simulink model "FREE_DRIFT"  (R2020b)
settings: Solver=ode4  StartTime=0.0  StopTime=500  FixedStep=Dt  RelTol=1e-3
values from neighbouring files (symbols this model uses):
  alpha = 0.01    [INPUTS_GRUPPO20.m]
  e_ss = 0.02    [INPUTS_GRUPPO20.m]
  enable_drag = 1    [INPUTS_GRUPPO20.m]
  enable_J2 = 1    [INPUTS_GRUPPO20.m]
  enable_Mgrav = 1    [INPUTS_GRUPPO20.m]
  enable_PD = 1    [INPUTS_GRUPPO20.m]
  enable_SMC = 0    [INPUTS_GRUPPO20.m]
  F_D = -1/2*rho*CD*A*Vx^2    (= -3.88125057814e-05)    [INPUTS_GRUPPO20.m]
  FJ2 = -3*J2*m_c0*mu*r_E^2/(2*r^4)    (= -0.00149705073945)    [INPUTS_GRUPPO20.m]
  gmax = 0.005    [INPUTS_GRUPPO20.m]
  INV_ZZZ = pinv(ZZZ)    [INPUTS_GRUPPO20.m]
  invJ = inv(J)    [INPUTS_GRUPPO20.m]
  J = J0    [INPUTS_GRUPPO20.m]
  kd = d*eye(3)    [INPUTS_GRUPPO20.m]
  kp1 = k*eye(3)    [INPUTS_GRUPPO20.m]
  Kr = 1    [INPUTS_GRUPPO20.m]
  lambda = 0.03    [INPUTS_GRUPPO20.m]
  m_c0 = 120    [INPUTS_GRUPPO20.m]
  omega = (mu/r^3)^0.5    (= 0.00113136572666)    [INPUTS_GRUPPO20.m]
  p_RW = 1    [INPUTS_GRUPPO20.m]
  Pos0 = Pos_RB(end,:)'    [INPUTS_GRUPPO20.m]
  q0_0 = Q_RB(end,1)'    [INPUTS_GRUPPO20.m]
  q_des = [1 0 0 0]'    [INPUTS_GRUPPO20.m]
  qv_0 = Q_RB(end,2:4)'    [INPUTS_GRUPPO20.m]
  tau_RW = 1.5645e-2    (= 0.015645)    [INPUTS_GRUPPO20.m]
  Vel0 = Vel_RB(end,:)'    [INPUTS_GRUPPO20.m]
  wb_0 = wb_RB(end,:)'    [INPUTS_GRUPPO20.m]
  X0_H = -10250    [INPUTS_GRUPPO20.m]
  ZZZ = [cos(B)    0      -cos(B)    0 ... (first row only)    [INPUTS_GRUPPO20.m]
undefined symbols (not defined in the file or in its folder): magnitude
libraries: vrlib x3, aerolibutil x1, sharedtransform x1
settings Model: Creator=Beniamino  LastModifiedBy=Beniamino

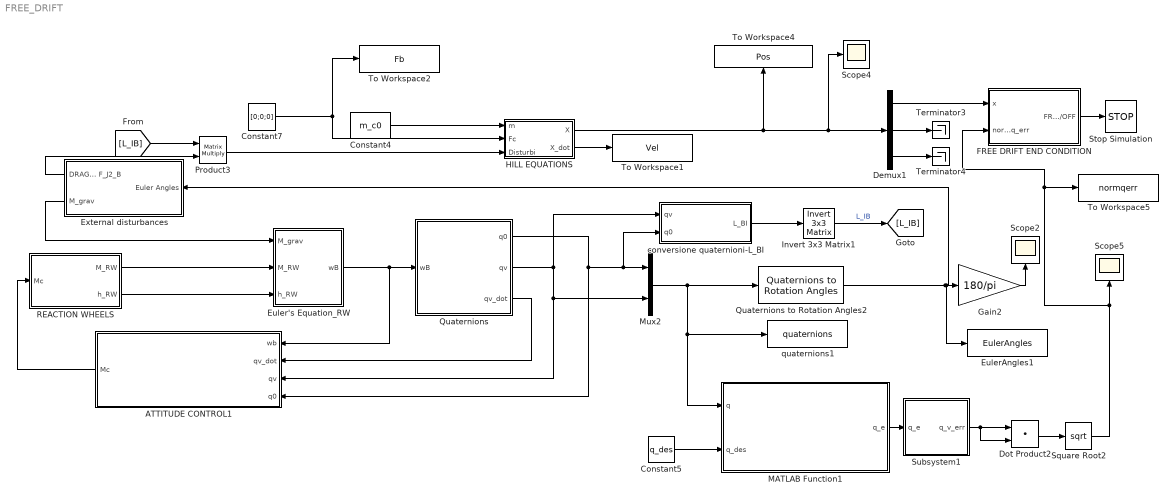
== system FREE_DRIFT ==
  ATTITUDE CONTROL1 : Subsystem
  Constant4 : Constant  Value=m_c0
  Constant5 : Constant  Value=q_des
  Constant7 : Constant  Value=[0;0;0]
  Demux1 : Demux  Outputs=3
  Dot Product2 : DotProduct  InputSameDT=on  OutDataTypeStr=Inherit: Inherit via internal rule
  Euler's Equation_RW : Subsystem
  EulerAngles1 : ToWorkspace  VariableName=EulerAngles  SampleTime=-1
  External disturbances : Subsystem
  FREE DRIFT END CONDITION : Subsystem
  Gain2 : Gain  Gain=180/pi
  HILL EQUATIONS : Subsystem
  Invert 3x3 Matrix1 : aerolibutil/Invert  3x3 Matrix
  MATLAB Function1 : MATLAB Function  TreatAsAtomicUnit=on
  Mux2 : Mux  Inputs=2
  Product3 : Product  Multiplication=Matrix(*)
  Quaternions : Subsystem
  Quaternions to Rotation Angles2 : sharedtransform/Quaternions to Rotation Angles  rotationOrder=ZYX  aMode=aMode
      settings: SourceProductBaseCode=AE,PW,MT,UV,VE,VP
  REACTION WHEELS : Subsystem
  Scope2 : Scope
  Scope4 : Scope
  Scope5 : Scope
  Square Root2 : Sqrt  SaturateOnIntegerOverflow=on
  Stop Simulation : Stop
  Subsystem1 : Subsystem
  Terminator3 : Terminator
  Terminator4 : Terminator
  To Workspace1 : ToWorkspace  VariableName=Vel  SampleTime=-1
  To Workspace2 : ToWorkspace  VariableName=Fb  SampleTime=-1
  To Workspace4 : ToWorkspace  VariableName=Pos  SampleTime=-1
  To Workspace5 : ToWorkspace  VariableName=normqerr  SampleTime=-1
  conversione quaternioni-L_BI : Subsystem
  quaternions1 : ToWorkspace  VariableName=quaternions  SampleTime=-1
  wires:
  External disturbances/2(M_grav) -> Euler's Equation_RW/1(M_grav)
  [L_IB] -> Product3/1
  Quaternions to Rotation Angles2/1 -> External disturbances/1(Euler Angles), EulerAngles1/1, Gain2/1
  REACTION WHEELS/2("h_RW ") -> Euler's Equation_RW/3(h_RW)
  Invert 3x3 Matrix1/1 -> [L_IB]  "L_IB"
  Product3/1 -> HILL EQUATIONS/3(Disturbi)
  Quaternions/1(q0) -> ATTITUDE CONTROL1/4(q0), Mux2/1, conversione quaternioni-L_BI/2(q0)
  Constant5/1 -> MATLAB Function1/2(q_des)
  Quaternions/3(qv_dot) -> ATTITUDE CONTROL1/2(qv_dot)
  External disturbances/1(DRAG_B + F_J2_B) -> Product3/2
  REACTION WHEELS/1(M_RW) -> Euler's Equation_RW/2(M_RW)
  Euler's Equation_RW/1(wB) -> ATTITUDE CONTROL1/1(wb), Quaternions/1(wB)
  MATLAB Function1/1(q_e) -> Subsystem1/1(q_e)
  Gain2/1 -> Scope2/1
  Subsystem1/1(q_v_err) -> Dot Product2/2, Dot Product2/1
  Quaternions/2(qv) -> ATTITUDE CONTROL1/3(qv), Mux2/2, conversione quaternioni-L_BI/1(qv)
  Mux2/1 -> Quaternions to Rotation Angles2/1, MATLAB Function1/1(q), quaternions1/1
  ATTITUDE CONTROL1/1(Mc) -> REACTION WHEELS/1(Mc)
  conversione quaternioni-L_BI/1(L_BI) -> Invert 3x3 Matrix1/1
  Dot Product2/1 -> Square Root2/1
  Constant7/1 -> HILL EQUATIONS/2(Fc), To Workspace2/1
  HILL EQUATIONS/2(X_dot) -> To Workspace1/1
  HILL EQUATIONS/1(X) -> Scope4/1, Demux1/1, To Workspace4/1
  Demux1/1 -> FREE DRIFT END CONDITION/1(x)
  Demux1/2 -> Terminator3/1
  Demux1/3 -> Terminator4/1
  Square Root2/1 -> To Workspace5/1, FREE DRIFT END CONDITION/2(norma q_err), Scope5/1
  FREE DRIFT END CONDITION/1(FREE DRIFT ON/OFF) -> Stop Simulation/1
  Constant4/1 -> HILL EQUATIONS/1(m)

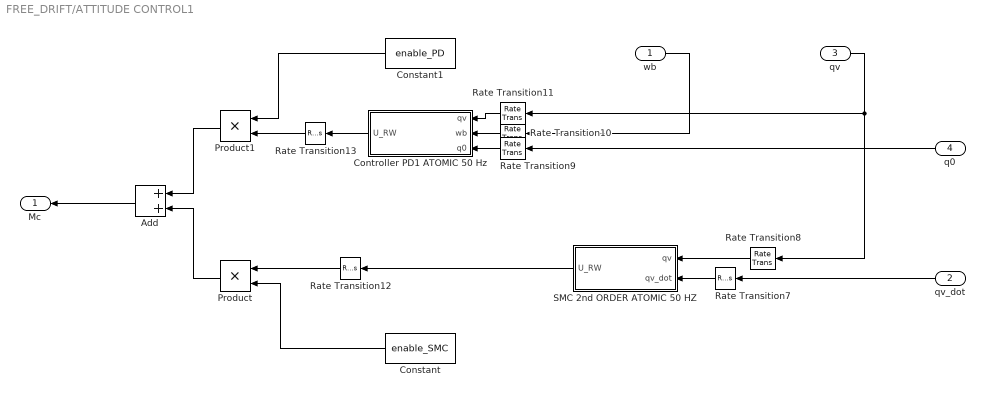
== system FREE_DRIFT/ATTITUDE CONTROL1 ==
  wb : Inport
  qv_dot : Inport  Port=2
  qv : Inport  Port=3
  q0 : Inport  Port=4
  Add : Sum
  Constant : Constant  Value=enable_SMC
  Constant1 : Constant  Value=enable_PD
  Controller PD1 ATOMIC 50 Hz : Subsystem  TreatAsAtomicUnit=on  SystemSampleTime=0.02
  Product : Product
  Product1 : Product
  Rate Transition{7..11} (5 alike) : RateTransition  OutPortSampleTime=Dt_con
  Rate Transition12 : RateTransition  OutPortSampleTime=Dt
  Rate Transition13 : RateTransition  OutPortSampleTime=Dt
  SMC 2nd ORDER ATOMIC 50 HZ : Subsystem  TreatAsAtomicUnit=on  SystemSampleTime=0.02
  Mc : Outport
  wires:
  Add/1 -> Mc/1
  qv_dot/1 -> Rate Transition7/1
  q0/1 -> Rate Transition9/1
  SMC 2nd ORDER ATOMIC 50 HZ/1(U_RW) -> Rate Transition12/1
  Controller PD1 ATOMIC 50 Hz/1(U_RW) -> Rate Transition13/1
  Rate Transition8/1 -> SMC 2nd ORDER ATOMIC 50 HZ/1(qv)
  wb/1 -> Rate Transition10/1
  Rate Transition7/1 -> SMC 2nd ORDER ATOMIC 50 HZ/2(qv_dot)
  Rate Transition10/1 -> Controller PD1 ATOMIC 50 Hz/2(wb)
  Rate Transition11/1 -> Controller PD1 ATOMIC 50 Hz/1(qv)
  qv/1 -> Rate Transition11/1, Rate Transition8/1
  Rate Transition9/1 -> Controller PD1 ATOMIC 50 Hz/3(q0)
  Rate Transition12/1 -> Product/1
  Constant/1 -> Product/2
  Rate Transition13/1 -> Product1/2
  Constant1/1 -> Product1/1
  Product1/1 -> Add/1
  Product/1 -> Add/2

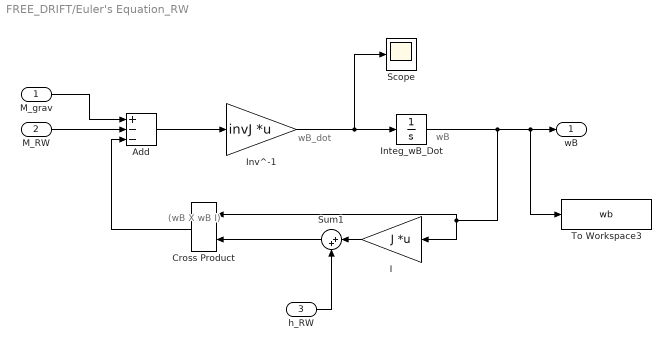
== system FREE_DRIFT/Euler's Equation_RW ==
  note: (wB X wB I)
  note: wB
  note: wB_dot
  M_grav : Inport
  M_RW : Inport  Port=2
  h_RW : Inport  Port=3
  Add : Sum  Inputs=+--
  Cross Product : vrlib/Utilities/Cross Product
  I : Gain  Gain=J  Multiplication=Matrix(K*u)
  Integ_wB_Dot : Integrator  InitialCondition=wb_0
  Inv^-1 : Gain  Gain=invJ  Multiplication=Matrix(K*u)
  Scope : Scope
  Sum1 : Sum  Inputs=|++
  To Workspace3 : ToWorkspace  VariableName=wb  SampleTime=-1
  wB : Outport  VectorParamsAs1DForOutWhenUnconnected=off
  wires:
  M_grav/1 -> Add/1
  Sum1/1 -> Cross Product/2
  h_RW/1 -> Sum1/2
  Integ_wB_Dot/1 -> To Workspace3/1, wB/1, Cross Product/1, I/1
  I/1 -> Sum1/1
  M_RW/1 -> Add/2
  Add/1 -> Inv^-1/1
  Inv^-1/1 -> Scope/1, Integ_wB_Dot/1
  Cross Product/1 -> Add/3

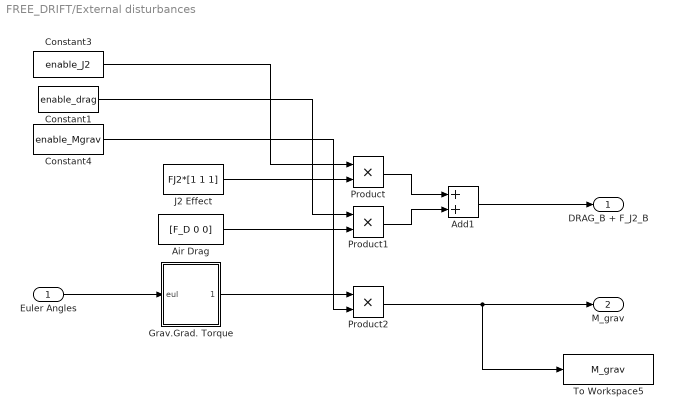
== system FREE_DRIFT/External disturbances ==
  Euler Angles : Inport
  Add1 : Sum
  Air Drag : Constant  Value=[F_D 0 0]
  Constant1 : Constant  Value=enable_drag
  Constant3 : Constant  Value=enable_J2
  Constant4 : Constant  Value=enable_Mgrav
  Grav.Grad. Torque : Subsystem
  J2 Effect : Constant  Value=FJ2*[1 1 1]
  Product : Product
  Product1 : Product
  Product2 : Product
  To Workspace5 : ToWorkspace  VariableName=M_grav  SampleTime=-1
  DRAG_B + F_J2_B : Outport
  M_grav : Outport  Port=2
  wires:
  Grav.Grad. Torque/1(M_grav) -> Product2/1
  Euler Angles/1 -> Grav.Grad. Torque/1(eul)
  Add1/1 -> DRAG_B + F_J2_B/1
  Constant3/1 -> Product/1
  J2 Effect/1 -> Product/2
  Constant1/1 -> Product1/1
  Air Drag/1 -> Product1/2
  Constant4/1 -> Product2/2
  Product/1 -> Add1/1
  Product1/1 -> Add1/2
  Product2/1 -> To Workspace5/1, M_grav/1

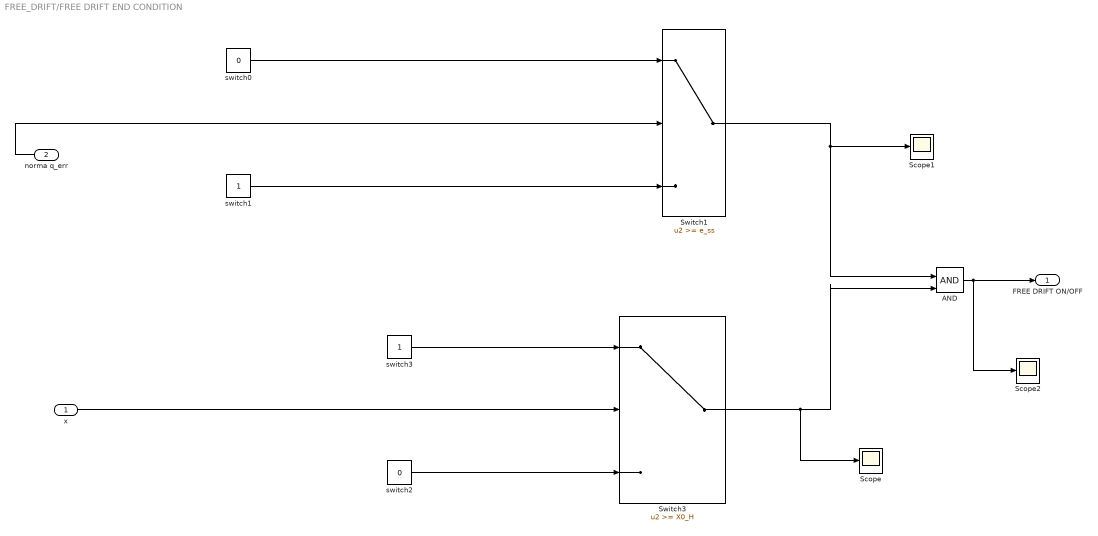
== system FREE_DRIFT/FREE DRIFT END CONDITION ==
  x : Inport
  norma q_err : Inport  Port=2
  AND : Logic  IconShape=distinctive  AllPortsSameDT=off  OutDataTypeStr=boolean
  Scope : Scope
  Scope1 : Scope
  Scope2 : Scope
  Switch1 : Switch  Threshold=e_ss
  Switch3 : Switch  Threshold=X0_H
  switch0 : Constant  Value=0
  switch1 : Constant
  switch2 : Constant  Value=0
  switch3 : Constant
  FREE DRIFT ON/OFF : Outport
  wires:
  norma q_err/1 -> Switch1/2
  Switch1/1 -> Scope1/1, AND/1
  switch0/1 -> Switch1/1
  switch2/1 -> Switch3/3
  Switch3/1 -> Scope/1, AND/2
  switch3/1 -> Switch3/1
  AND/1 -> Scope2/1, FREE DRIFT ON/OFF/1
  switch1/1 -> Switch1/3
  x/1 -> Switch3/2

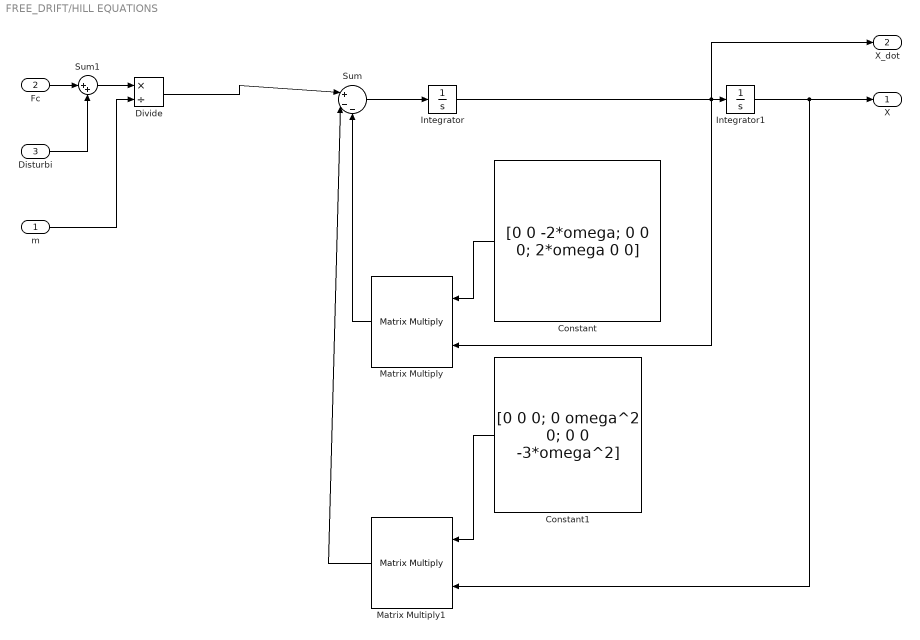
== system FREE_DRIFT/HILL EQUATIONS ==
  m : Inport
  Fc : Inport  Port=2
  Disturbi : Inport  Port=3
  Constant : Constant  Value=[0 0 -2*omega; 0 0 0; 2*omega 0 0]
  Constant1 : Constant  Value=[0 0 0; 0 omega^2 0; 0 0 -3*omega^2]
  Divide : Product  Inputs=*/
  Integrator : Integrator  InitialCondition=Vel0
  Integrator1 : Integrator  InitialCondition=Pos0
  Matrix Multiply : Product  Multiplication=Matrix(*)
  Matrix Multiply1 : Product  Multiplication=Matrix(*)
  Sum : Sum  Inputs=|+--
  Sum1 : Sum  Inputs=|++
  X : Outport
  X_dot : Outport  Port=2
  wires:
  Constant/1 -> Matrix Multiply/1
  Sum1/1 -> Divide/1
  Disturbi/1 -> Sum1/2
  Integrator/1 -> Integrator1/1, X_dot/1, Matrix Multiply/2
  Fc/1 -> Sum1/1
  m/1 -> Divide/2
  Matrix Multiply1/1 -> Sum/2
  Matrix Multiply/1 -> Sum/3
  Constant1/1 -> Matrix Multiply1/1
  Integrator1/1 -> Matrix Multiply1/2, X/1
  Sum/1 -> Integrator/1
  Divide/1 -> Sum/1

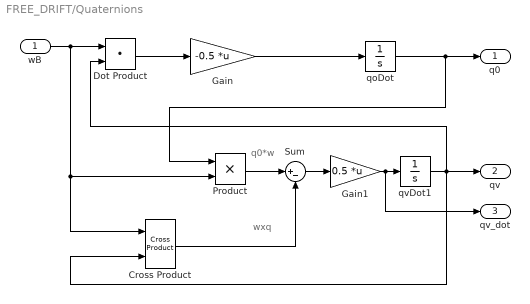
== system FREE_DRIFT/Quaternions ==
  note: wxq
  note: q0*w
  wB : Inport
  Cross Product : vrlib/Utilities/Cross Product
  Dot Product : DotProduct  InputSameDT=on  OutDataTypeStr=Inherit: Inherit via internal rule
  Gain : Gain  Gain=-0.5  Multiplication=Matrix(K*u)
  Gain1 : Gain  Gain=0.5  Multiplication=Matrix(K*u)
  Product : Product  RndMeth=Zero
  Sum : Sum  Inputs=|+-
  qoDot : Integrator  InitialCondition=q0_0
  qvDot1 : Integrator  InitialCondition=qv_0
  q0 : Outport  VectorParamsAs1DForOutWhenUnconnected=off
  qv : Outport  Port=2  VectorParamsAs1DForOutWhenUnconnected=off
  qv_dot : Outport  Port=3  VectorParamsAs1DForOutWhenUnconnected=off
  wires:
  qoDot/1 -> q0/1, Product/1
  qvDot1/1 -> Cross Product/2, qv/1, Dot Product/2
  wB/1 -> Cross Product/1, Product/2, Dot Product/1
  Dot Product/1 -> Gain/1
  Gain/1 -> qoDot/1
  Product/1 -> Sum/1
  Cross Product/1 -> Sum/2
  Sum/1 -> Gain1/1
  Gain1/1 -> qvDot1/1, qv_dot/1

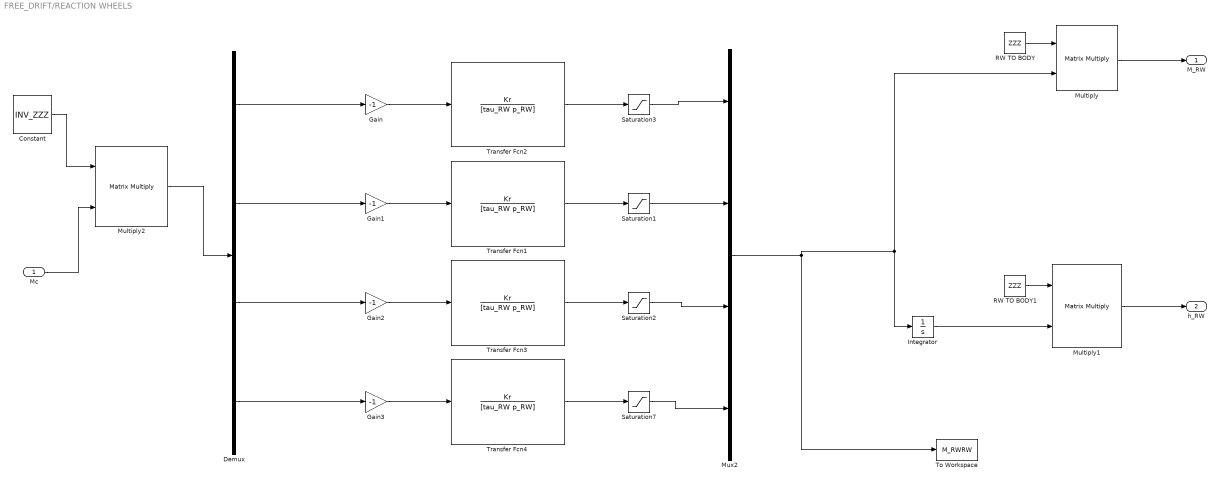
== system FREE_DRIFT/REACTION WHEELS ==
  Mc : Inport
  Constant : Constant  Value=INV_ZZZ
  Demux : Demux
  Gain{,1..3} (4 alike) : Gain  Gain=-1
  Integrator : Integrator
  Multiply : Product  Multiplication=Matrix(*)
  Multiply1 : Product  Multiplication=Matrix(*)
  Multiply2 : Product  Multiplication=Matrix(*)
  Mux2 : Mux
  RW TO BODY : Constant  Value=ZZZ
  RW TO BODY1 : Constant  Value=ZZZ
  Saturation{1..3,7} (4 alike) : Saturate  UpperLimit=gmax  LowerLimit=-gmax
  To Workspace : ToWorkspace  VariableName=M_RWRW  SampleTime=-1
  Transfer Fcn{1..4} (4 alike) : TransferFcn  Numerator=Kr  Denominator=[tau_RW p_RW]
  M_RW : Outport  VectorParamsAs1DForOutWhenUnconnected=off
  "h_RW " : Outport  Port=2  VectorParamsAs1DForOutWhenUnconnected=off
  wires:
  Mc/1 -> Multiply2/2
  Multiply/1 -> M_RW/1
  Demux/1 -> Gain/1
  Demux/2 -> Gain1/1
  Demux/3 -> Gain2/1
  Gain/1 -> Transfer Fcn2/1
  Gain1/1 -> Transfer Fcn1/1
  Gain2/1 -> Transfer Fcn3/1
  Multiply1/1 -> "h_RW "/1
  Demux/4 -> Gain3/1
  Gain3/1 -> Transfer Fcn4/1
  RW TO BODY/1 -> Multiply/1
  RW TO BODY1/1 -> Multiply1/1
  Constant/1 -> Multiply2/1
  Multiply2/1 -> Demux/1
  Transfer Fcn4/1 -> Saturation7/1
  Mux2/1 -> To Workspace/1, Multiply/2, Integrator/1
  Integrator/1 -> Multiply1/2
  Saturation7/1 -> Mux2/4
  Transfer Fcn3/1 -> Saturation2/1
  Saturation2/1 -> Mux2/3
  Transfer Fcn1/1 -> Saturation1/1
  Saturation1/1 -> Mux2/2
  Transfer Fcn2/1 -> Saturation3/1
  Saturation3/1 -> Mux2/1

== system FREE_DRIFT/Subsystem1 ==
  q_e : Inport
  Demux : Demux
  Mux1 : Mux  Inputs=3
  Terminator : Terminator
  q_v_err : Outport  VectorParamsAs1DForOutWhenUnconnected=off
  wires:
  Demux/3 -> Mux1/2
  Demux/2 -> Mux1/1
  Demux/4 -> Mux1/3
  Demux/1 -> Terminator/1
  q_e/1 -> Demux/1
  Mux1/1 -> q_v_err/1

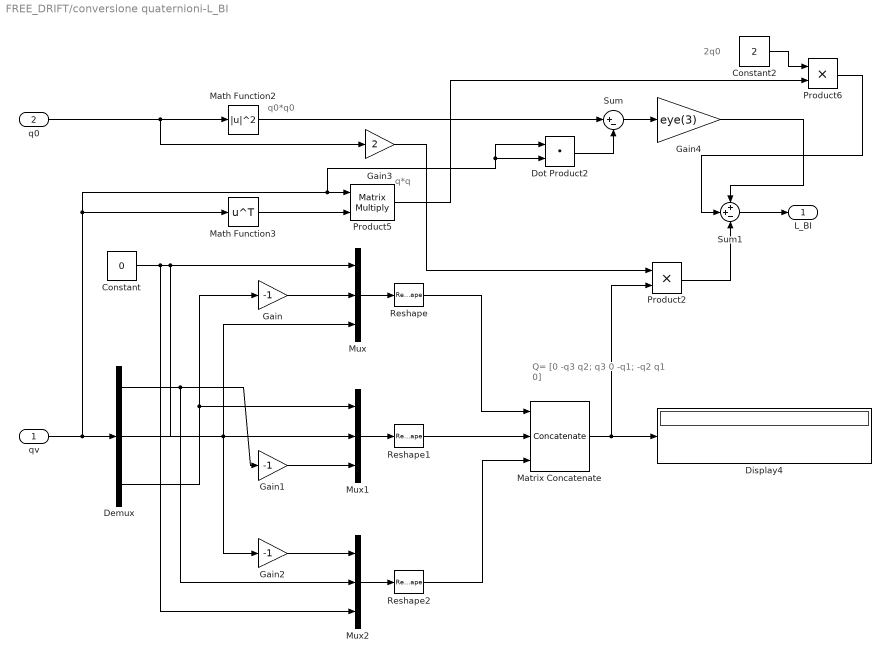
== system FREE_DRIFT/conversione quaternioni-L_BI ==
  note: Q= [0 -q3 q2;
      | 	q3 0 -q1;
      | 	-q2 q1 0]
  note: 2q0
  note: q*q
  note: q0*q0
  qv : Inport
  q0 : Inport  Port=2
  Constant : Constant  Value=0
  Constant2 : Constant  Value=2
  Demux : Demux  Outputs=3
  Display4 : Display
  Dot Product2 : DotProduct  InputSameDT=on  OutDataTypeStr=Inherit: Inherit via internal rule
  Gain : Gain  Gain=-1
  Gain1 : Gain  Gain=-1
  Gain2 : Gain  Gain=-1
  Gain3 : Gain  Gain=2
  Gain4 : Gain  Gain=eye(3)
  Math Function2 : Math  Operator=magnitude^2  SignedPower=on  SaturateOnIntegerOverflow=on
  Math Function3 : Math  Operator=transpose  SignedPower=on  SaturateOnIntegerOverflow=on
  Matrix Concatenate : Concatenate  NumInputs=3  Mode=Multidimensional array
  Mux : Mux  Inputs=3
  Mux1 : Mux  Inputs=3
  Mux2 : Mux  Inputs=3
  Product2 : Product  RndMeth=Zero
  Product5 : Product  Multiplication=Matrix(*)
  Product6 : Product
  Reshape : Reshape  OutputDimensionality=Row vector (2-D)
  Reshape1 : Reshape  OutputDimensionality=Row vector (2-D)
  Reshape2 : Reshape  OutputDimensionality=Row vector (2-D)
  Sum : Sum  Inputs=|+-
  Sum1 : Sum  Inputs=++-
  L_BI : Outport  VectorParamsAs1DForOutWhenUnconnected=off
  wires:
  qv/1 -> Demux/1, Product5/1, Dot Product2/2, Dot Product2/1, Math Function3/1
  Constant/1 -> Mux/1, Mux1/2, Mux2/3
  Demux/3 -> Gain/1, Mux1/1
  Gain/1 -> Mux/2
  Demux/2 -> Mux/3, Gain2/1
  Gain1/1 -> Mux1/3
  Demux/1 -> Gain1/1, Mux2/2
  Gain2/1 -> Mux2/1
  q0/1 -> Gain3/1, Math Function2/1
  Math Function2/1 -> Sum/1
  Gain4/1 -> Sum1/1
  Product6/1 -> Sum1/2
  Product2/1 -> Sum1/3
  Sum1/1 -> L_BI/1
  Matrix Concatenate/1 -> Product2/2, Display4/1
  Mux/1 -> Reshape/1
  Reshape/1 -> Matrix Concatenate/1
  Mux2/1 -> Reshape2/1
  Reshape2/1 -> Matrix Concatenate/3
  Mux1/1 -> Reshape1/1
  Reshape1/1 -> Matrix Concatenate/2
  Sum/1 -> Gain4/1
  Math Function3/1 -> Product5/2
  Gain3/1 -> Product2/1
  Product5/1 -> Product6/2
  Constant2/1 -> Product6/1
  Dot Product2/1 -> Sum/2

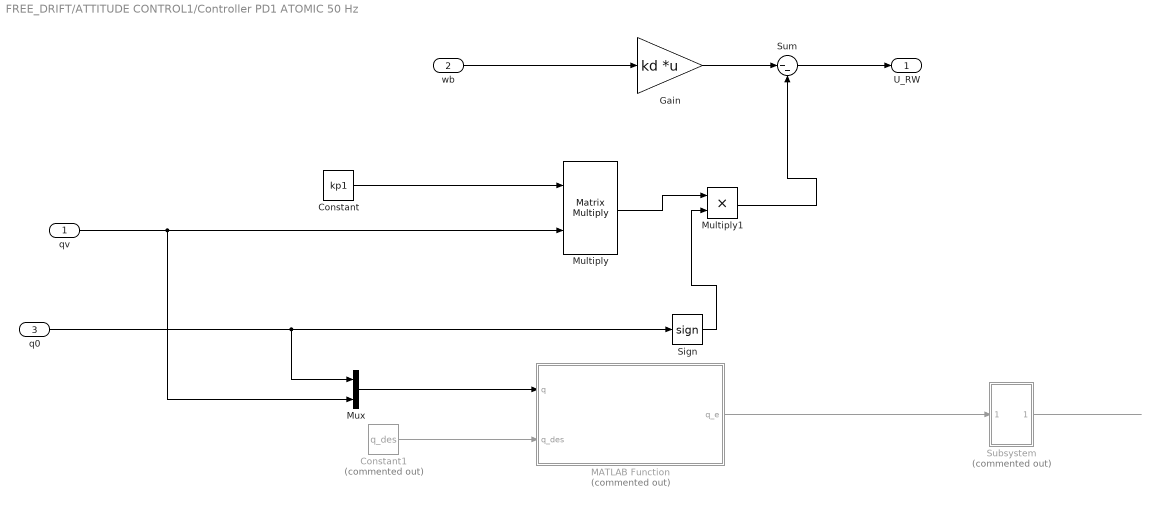
== system FREE_DRIFT/ATTITUDE CONTROL1/Controller PD1 ATOMIC 50 Hz ==
  qv : Inport
  wb : Inport  Port=2
  q0 : Inport  Port=3
  Constant : Constant  Value=kp1
  Constant1 : Constant  Commented=on  Value=q_des
  Gain : Gain  Gain=kd  Multiplication=Matrix(K*u) (u vector)
  MATLAB Function : MATLAB Function  Commented=on  TreatAsAtomicUnit=on
  Multiply : Product  Multiplication=Matrix(*)
  Multiply1 : Product
  Mux : Mux  Inputs=2
  Sign : Signum
  Subsystem : Subsystem  Commented=on
  Sum : Sum  Inputs=|--
  U_RW : Outport  VectorParamsAs1DForOutWhenUnconnected=off
  wires:
  Constant1/1 -> MATLAB Function/2(q_des)
  Gain/1 -> Sum/1
  Constant/1 -> Multiply/1
  Mux/1 -> MATLAB Function/1(q)
  q0/1 -> Mux/1, Sign/1
  Multiply/1 -> Multiply1/1
  wb/1 -> Gain/1
  MATLAB Function/1(q_e) -> Subsystem/1(q_e)
  Sign/1 -> Multiply1/2
  Multiply1/1 -> Sum/2
  Sum/1 -> U_RW/1
  qv/1 -> Mux/2, Multiply/2
  Subsystem/1(q_err) -> ?

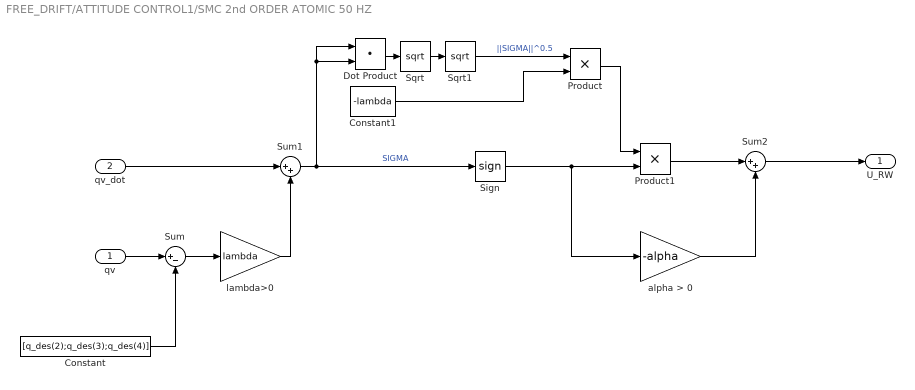
== system FREE_DRIFT/ATTITUDE CONTROL1/SMC 2nd ORDER ATOMIC 50 HZ ==
  qv : Inport
  qv_dot : Inport  Port=2
  Constant : Constant  Value=[q_des(2);q_des(3);q_des(4)]
  Constant1 : Constant  Value=-lambda
  Dot Product : DotProduct  InputSameDT=on  OutDataTypeStr=Inherit: Inherit via internal rule
  Product : Product
  Product1 : Product
  Sign : Signum
  Sqrt : Sqrt  SaturateOnIntegerOverflow=on
  Sqrt1 : Sqrt  SaturateOnIntegerOverflow=on
  Sum : Sum  Inputs=|+-
  Sum1 : Sum  Inputs=|++
  Sum2 : Sum  Inputs=|++
  alpha > 0 : Gain  Gain=-alpha
  lambda>0 : Gain  Gain=lambda
  U_RW : Outport
  wires:
  Constant1/1 -> Product/2
  alpha > 0/1 -> Sum2/2
  Product1/1 -> Sum2/1
  Dot Product/1 -> Sqrt/1
  Sum/1 -> lambda>0/1
  Sum2/1 -> U_RW/1
  Product/1 -> Product1/1
  Sign/1 -> alpha > 0/1, Product1/2
  lambda>0/1 -> Sum1/2
  Constant/1 -> Sum/2
  Sum1/1 -> Sign/1, Dot Product/1, Dot Product/2  "SIGMA"
  Sqrt/1 -> Sqrt1/1
  Sqrt1/1 -> Product/1  "||SIGMA||^0.5"
  qv_dot/1 -> Sum1/1
  qv/1 -> Sum/1

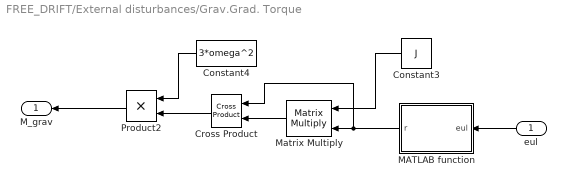
== system FREE_DRIFT/External disturbances/Grav.Grad. Torque ==
  eul : Inport
  Constant3 : Constant  Value=J
  Constant4 : Constant  Value=3*omega^2
  Cross Product : vrlib/Utilities/Cross Product
  MATLAB function : MATLAB Function  TreatAsAtomicUnit=on
  Matrix Multiply : Product  Multiplication=Matrix(*)
  Product2 : Product
  M_grav : Outport
  wires:
  Constant3/1 -> Matrix Multiply/1
  MATLAB function/1(r) -> Matrix Multiply/2, Cross Product/1
  Cross Product/1 -> Product2/2
  Constant4/1 -> Product2/1
  Product2/1 -> M_grav/1
  eul/1 -> MATLAB function/1(eul)
  Matrix Multiply/1 -> Cross Product/2

== system FREE_DRIFT/ATTITUDE CONTROL1/Controller PD1 ATOMIC 50 Hz/Subsystem ==
  q_e : Inport
  Demux : Demux
  Mux1 : Mux  Inputs=3
  Terminator : Terminator
  q_err : Outport  VectorParamsAs1DForOutWhenUnconnected=off
  wires:
  Demux/3 -> Mux1/2
  Demux/2 -> Mux1/1
  Demux/4 -> Mux1/3
  Demux/1 -> Terminator/1
  q_e/1 -> Demux/1
  Mux1/1 -> q_err/1

== matlab function FREE_DRIFT/ATTITUDE CONTROL1/Controller PD1 ATOMIC 50 Hz/MATLAB Function ==
  data: q input; q_e output; q_des input
function q_e = quaternion_error(q, q_des)
%#codegen

q_inv = [q_des(1) -q_des(2) -q_des(3) -q_des(4)]'/(q_des(1)^2+q_des(2)^2 + q_des(3)^2+q_des(4)^2);

Q   = [q_inv(1) -q_inv(2) -q_inv(3) -q_inv(4)
       q_inv(2)  q_inv(1) -q_inv(4)  q_inv(3)
       q_inv(3)  q_inv(4)  q_inv(1) -q_inv(2)
       q_inv(4) -q_inv(3)  q_inv(2)  q_inv(1)];
q_e =Q*q;

== matlab function FREE_DRIFT/External disturbances/Grav.Grad. Torque/MATLAB function ==
  data: eul input; r output
function r = fcn(eul)
    r = [-sin(eul(2)); sin(eul(3)); 1-(sin(eul(2)))^2-(sin(eul(3)))^2];

== matlab function FREE_DRIFT/MATLAB Function1 ==
  data: q input; q_e output; q_des input
function q_e = quaternion_error(q, q_des)
%#codegen

q_inv = [q_des(1) -q_des(2) -q_des(3) -q_des(4)]'/(q_des(1)^2+q_des(2)^2 + q_des(3)^2+q_des(4)^2);

Q   = [q_inv(1) -q_inv(2) -q_inv(3) -q_inv(4)
       q_inv(2)  q_inv(1) -q_inv(4)  q_inv(3)
       q_inv(3)  q_inv(4)  q_inv(1) -q_inv(2)
       q_inv(4) -q_inv(3)  q_inv(2)  q_inv(1)];
q_e =Q*q;
